simulink model "tank"  (Simulink 3.00)
settings: Solver=ode45  StartTime=0.0  StopTime=200.0  RelTol=1e-5
values from neighbouring files (symbols this model uses):
  conegain = 1/(tan(conealpha*pi/180)^2*pi)    [simparam.m]
  kout = 0.0001    [simparam.m]
  starth = 0.1    [simparam.m]
settings Model: Creator=pmn  LastModifiedBy=pmn

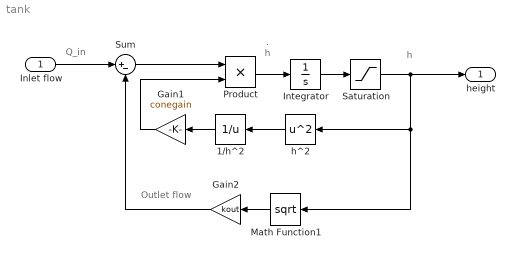
== system tank ==
  note: h
  note: h
  note: .
  note: Q_in
  note: Outlet flow
  Inlet flow : Inport  Port=1  PortWidth=-1  SampleTime=-1  DataType=auto
      settings: SignalType=auto
  1/h^2 : Math  Orientation=left  Operator=reciprocal  OutputSignalType=auto
  Gain1 : Gain  Orientation=left  Gain=conegain  SaturateOnIntegerOverflow=off
  Gain2 : Gain  Orientation=left  Gain=kout  SaturateOnIntegerOverflow=off
  Integrator : Integrator  ExternalReset=none  InitialConditionSource=internal  InitialCondition=starth  LimitOutput=off  UpperSaturationLimit=inf  LowerSaturationLimit=-inf  ShowSaturationPort=off  ShowStatePort=off  AbsoluteTolerance=auto
  Math Function1 : Math  Orientation=left  Operator=sqrt  OutputSignalType=auto
  Product : Product  Inputs=2  SaturateOnIntegerOverflow=on
  Saturation : Saturate  UpperLimit=0.5  LowerLimit=1e-3
  Sum : Sum  Inputs=|+-  SaturateOnIntegerOverflow=on
  h^2 : Math  Orientation=left  Operator=square  OutputSignalType=auto
  height : Outport  Port=1
  wires:
  Gain2/1 -> Sum/2
  Math Function1/1 -> Gain2/1
  Product/1 -> Integrator/1
  Gain1/1 -> Product/2
  h^2/1 -> 1/h^2/1
  1/h^2/1 -> Gain1/1
  Sum/1 -> Product/1
  Integrator/1 -> Saturation/1
  Saturation/1 -> height/1, Math Function1/1, h^2/1
  Inlet flow/1 -> Sum/1
